simulink model "ZeroCrossDetection"  (R2022b)
settings: Solver=VariableStepAuto  StartTime=0.0  StopTime=0.08  MaxStep=1e-3  RelTol=1e-3
libraries: simulink x2
settings Model: Creator=Mo_7atem  LastModifiedBy=Mo_7atem

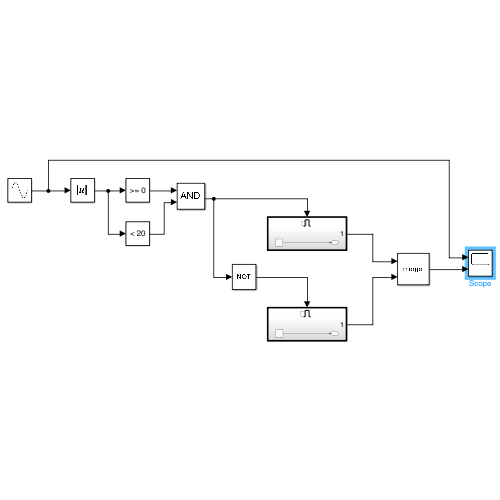
[thumbnail: Simulink's stored preview of the top-level diagram]
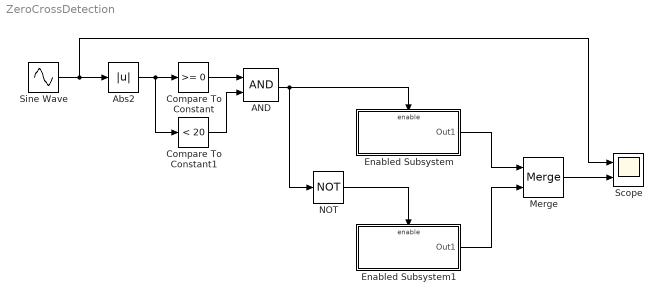
== system ZeroCrossDetection ==
  AND : Logic  AllPortsSameDT=off  OutDataTypeStr=boolean
  Abs2 : Abs  SaturateOnIntegerOverflow=off
  Compare To Constant : simulink/Logic and Bit Operations/Compare To Constant  relop=>=  const=0  OutDataTypeStr=boolean
  Compare To Constant1 : simulink/Logic and Bit Operations/Compare To Constant  relop=<  const=20  OutDataTypeStr=boolean  ZeroCross=off
  Enabled Subsystem : Subsystem  TreatAsAtomicUnit=on
  Enabled Subsystem1 : Subsystem  TreatAsAtomicUnit=on
  Merge : Merge
  NOT : Logic  Operator=NOT  AllPortsSameDT=off  OutDataTypeStr=boolean
  Scope : Scope  NumInputPorts=2
  Sine Wave : Sin  Amplitude=220  Frequency=2*pi*50  SampleTime=0
  wires:
  Compare To Constant/1 -> AND/1
  Compare To Constant1/1 -> AND/2
  AND/1 -> NOT/1, Enabled Subsystem/Enable
  NOT/1 -> Enabled Subsystem1/Enable
  Enabled Subsystem/1(Out1) -> Merge/1
  Enabled Subsystem1/1(Out1) -> Merge/2
  Merge/1 -> Scope/2
  Sine Wave/1 -> Abs2/1, Scope/1
  Abs2/1 -> Compare To Constant/1, Compare To Constant1/1

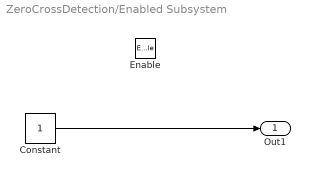
== system ZeroCrossDetection/Enabled Subsystem ==
  Enable : EnablePort
  Constant : Constant
  Out1 : Outport
  wires:
  Constant/1 -> Out1/1

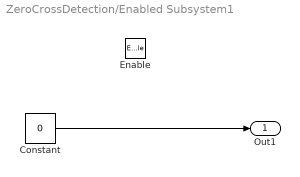
== system ZeroCrossDetection/Enabled Subsystem1 ==
  Enable : EnablePort
  Constant : Constant  Value=0
  Out1 : Outport
  wires:
  Constant/1 -> Out1/1
